simulink model "escestimatorfinal"  (R2021a)
settings: Solver=VariableStepAuto  StartTime=0.0  StopTime=10.0  RelTol=1e-3
values from neighbouring files (symbols this model uses):
  B = 18    [fourwheelvdmodelparam.m]
  C = 1.5    [fourwheelvdmodelparam.m]
  C_A = 0.5    [fourwheelvdmodelparam.m]
  Cr = 5800    [fourwheelvdmodelparam.m]
  Cy = 95000    [fourwheelvdmodelparam.m]
  D = 2000    [fourwheelvdmodelparam.m]
  g = 9.81    [fourwheelvdmodelparam.m]
  hs = 0.5    [fourwheelvdmodelparam.m]
  J = (0.5*(lf+lr))^2*m    (= 3825)    [fourwheelvdmodelparam.m]
  Jx = 800    [fourwheelvdmodelparam.m]
  K = 42000    [fourwheelvdmodelparam.m]
  lf = 1.5    [fourwheelvdmodelparam.m]
  lr = 1.5    [fourwheelvdmodelparam.m]
  m = 1700    [fourwheelvdmodelparam.m]
undefined symbols (not defined in the file or in its folder): Cx, Sfl, Sfr, Srl, Srr
libraries: simulink x2
settings Model: Creator=s361515  LastModifiedBy=s361515

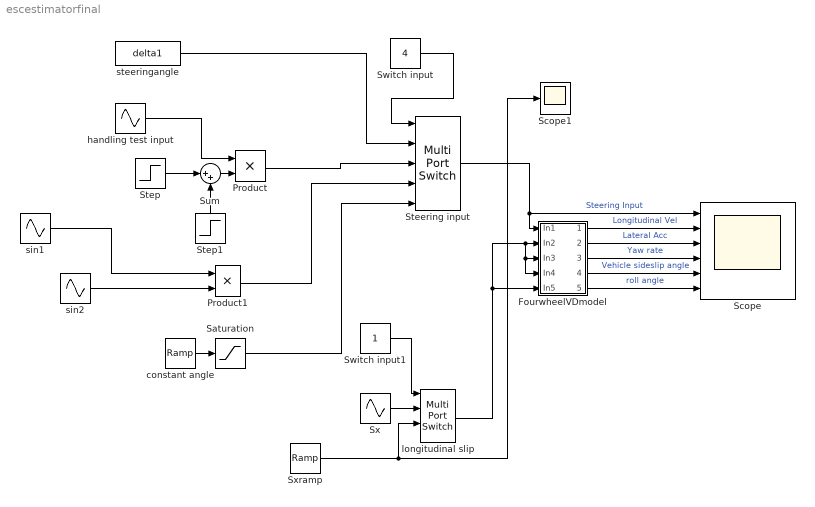
== system escestimatorfinal ==
  FourwheelVDmodel : Subsystem
  Product : Product
  Product1 : Product
  Saturation : Saturate  UpperLimit=5  LowerLimit=0
  Scope : Scope  NumInputPorts=6
  Scope1 : Scope
  Steering input : MultiPortSwitch  Inputs=4
  Step : Step  Time=1.5  SampleTime=0
  Step1 : Step  Time=8.5  After=-1  SampleTime=0
  Sum : Sum  Inputs=|++
  Switch input : Constant  Value=4
  Switch input1 : Constant
  Sx : Sin  Amplitude=0.5e-1  Bias=1.5e-1  Frequency=5*pi  SampleTime=0
  Sxramp : simulink/Sources/Ramp  slope=0.1  start=0  InitialOutput=0
  constant angle : simulink/Sources/Ramp  slope=1.5  start=0  InitialOutput=0
  handling test input : Sin  Amplitude=6  Frequency=pi  Phase=pi/2  SampleTime=0
  longitudinal slip : MultiPortSwitch
  sin1 : Sin  Amplitude=6  Frequency=pi/8  SampleTime=0
  sin2 : Sin  Frequency=pi  Phase=pi/2  SampleTime=0
  steeringangle : FromWorkspace  VariableName=delta1
  wires:
  sin1/1 -> Product1/1
  Product1/1 -> Steering input/4
  longitudinal slip/1 -> FourwheelVDmodel/5(In5), FourwheelVDmodel/4(In4), FourwheelVDmodel/3(In3), FourwheelVDmodel/2(In2)
  Switch input1/1 -> longitudinal slip/1
  Sxramp/1 -> Scope1/1, longitudinal slip/3
  sin2/1 -> Product1/2
  Step/1 -> Sum/1
  Step1/1 -> Sum/2
  handling test input/1 -> Product/1
  FourwheelVDmodel/1(Out1) -> Scope/2  "Longitudinal Vel"
  Product/1 -> Steering input/3
  FourwheelVDmodel/2(Out2) -> Scope/3  "Lateral Acc"
  Steering input/1 -> FourwheelVDmodel/1(In1), Scope/1  "Steering Input"
  Sum/1 -> Product/2
  constant angle/1 -> Saturation/1
  Sx/1 -> longitudinal slip/2
  FourwheelVDmodel/3(Out3) -> Scope/4  "Yaw rate"
  Switch input/1 -> Steering input/1
  FourwheelVDmodel/5(Out5) -> Scope/6  "roll angle"
  FourwheelVDmodel/4(Out4) -> Scope/5  "Vehicle sideslip angle"
  Saturation/1 -> Steering input/5
  steeringangle/1 -> Steering input/2

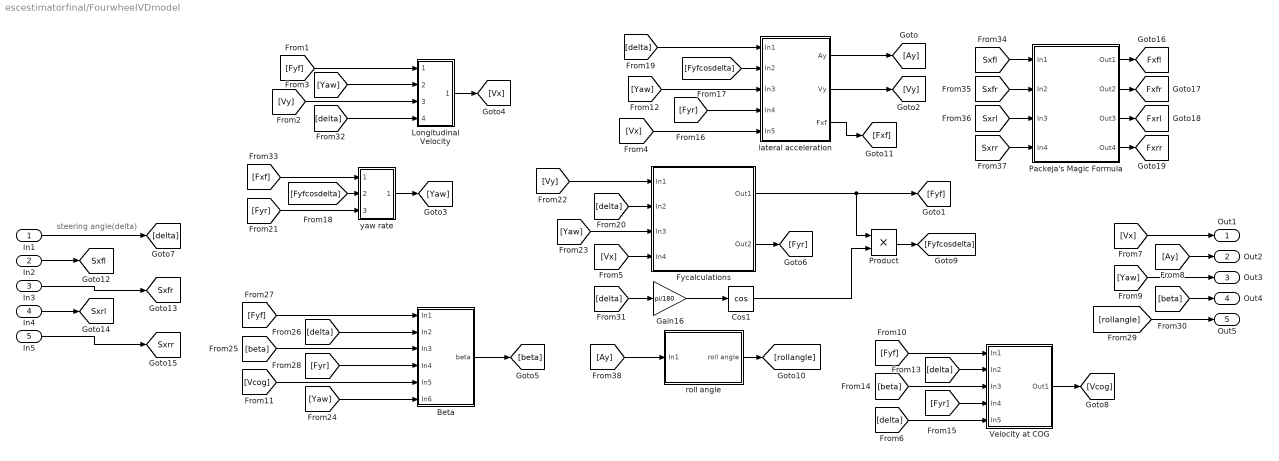
== system escestimatorfinal/FourwheelVDmodel ==
  note: steering angle(delta)
  In1 : Inport
  In2 : Inport  Port=2
  In3 : Inport  Port=3
  In4 : Inport  Port=4
  In5 : Inport  Port=5
  Beta : Subsystem
  Cos1 : Trigonometry  Operator=cos
  Fycalculations : Subsystem
  Gain16 : Gain  Gain=pi/180
  Longitudinal Velocity : Subsystem
  Packeja's Magic Formula : Subsystem
  Product : Product
  Velocity at COG : Subsystem
  lateral acceleration : Subsystem
  roll angle : Subsystem
  yaw rate : Subsystem
  Out1 : Outport
  Out2 : Outport  Port=2
  Out3 : Outport  Port=3
  Out4 : Outport  Port=4
  Out5 : Outport  Port=5
  tag scope: Fxfl=global, Fxfr=global, Fxrl=global, Fxrr=global, Sxfl=global, Sxfr=global, Sxrl=global, Sxrr=global
  wires:
  Gain16/1 -> Cos1/1
  Product/1 -> [Fyfcosdelta]
  In1/1 -> [delta]
  Cos1/1 -> Product/2
  [Vx] -> Out1/1
  [Ay] -> Out2/1
  [Yaw] -> Out3/1
  Longitudinal Velocity/1(Out1) -> [Vx]
  [Fyf] -> Longitudinal Velocity/1(In1)
  [Yaw] -> Longitudinal Velocity/2(In2)
  [Vy] -> Longitudinal Velocity/3(In3)
  lateral acceleration/2(Vy) -> [Vy]
  [Vx] -> lateral acceleration/5(In5)
  lateral acceleration/1(Ay) -> [Ay]
  [Yaw] -> lateral acceleration/3(In3)
  [Fyr] -> lateral acceleration/4(In4)
  [Fyfcosdelta] -> lateral acceleration/2(In2)
  [delta] -> lateral acceleration/1(In1)
  yaw rate/1(Out1) -> [Yaw]
  [Fyfcosdelta] -> yaw rate/2(In2)
  [Fyr] -> yaw rate/3(In3)
  Fycalculations/1(Out1) -> [Fyf], Product/1
  Fycalculations/2(Out2) -> [Fyr]
  [Vy] -> Fycalculations/1(In1)
  [delta] -> Fycalculations/2(In2)
  [Yaw] -> Fycalculations/3(In3)
  [Vx] -> Fycalculations/4(In4)
  Beta/1(beta) -> [beta]
  [Fyf] -> Beta/1(In1)
  [delta] -> Beta/2(In2)
  [beta] -> Beta/3(In3)
  [Fyr] -> Beta/4(In4)
  [Vcog] -> Beta/5(In5)
  [Yaw] -> Beta/6(In6)
  [Ay] -> roll angle/1(In1)
  roll angle/1(roll angle) -> [rollangle]
  [rollangle] -> Out5/1
  [beta] -> Out4/1
  [Fyf] -> Velocity at COG/1(In1)
  [delta] -> Velocity at COG/2(In2)
  [beta] -> Velocity at COG/3(In3)
  [Fyr] -> Velocity at COG/4(In4)
  [delta] -> Velocity at COG/5(In5)
  Velocity at COG/1(Out1) -> [Vcog]
  [delta] -> Gain16/1
  [delta] -> Longitudinal Velocity/4(In4)
  lateral acceleration/3(Fxf) -> [Fxf]
  [Fxf] -> yaw rate/1(In1)
  In5/1 -> [Sxrr]
  In4/1 -> [Sxrl]
  In3/1 -> [Sxfr]
  In2/1 -> [Sxfl]
  [Sxfl] -> Packeja's Magic Formula/1(In1)
  [Sxfr] -> Packeja's Magic Formula/2(In2)
  [Sxrl] -> Packeja's Magic Formula/3(In3)
  [Sxrr] -> Packeja's Magic Formula/4(In4)
  Packeja's Magic Formula/1(Out1) -> [Fxfl]
  Packeja's Magic Formula/4(Out4) -> [Fxrr]
  Packeja's Magic Formula/3(Out3) -> [Fxrl]
  Packeja's Magic Formula/2(Out2) -> [Fxfr]

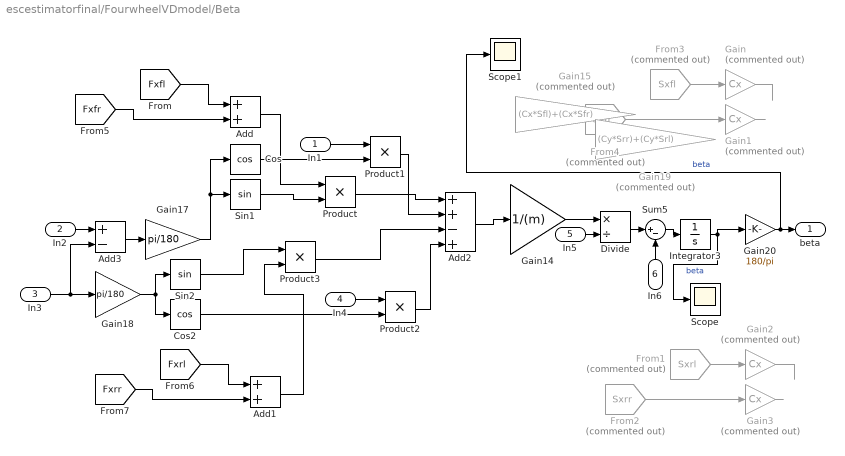
== system escestimatorfinal/FourwheelVDmodel/Beta ==
  In1 : Inport
  In2 : Inport  Port=2
  In3 : Inport  Port=3
  In4 : Inport  Port=4
  In5 : Inport  Port=5
  In6 : Inport  Port=6
  Add : Sum
  Add1 : Sum
  Add2 : Sum  Inputs=++-+
  Add3 : Sum  Inputs=+-
  Cos : Trigonometry  Operator=cos
  Cos2 : Trigonometry  Operator=cos
  Divide : Product  Inputs=*/
  From1 : From  Commented=on  GotoTag=Sxrl  TagVisibility=global
  From2 : From  Commented=on  GotoTag=Sxrr  TagVisibility=global
  From3 : From  Commented=on  GotoTag=Sxfl  TagVisibility=global
  From4 : From  Commented=on  GotoTag=Sxfr  TagVisibility=global
  Gain{,1..3} (4 alike) : Gain  Commented=on  Gain=Cx
  Gain14 : Gain  Gain=1/(m)
  Gain15 : Gain  Commented=on  Gain=(Cx*Sfl)+(Cx*Sfr)
  Gain17 : Gain  Gain=pi/180
  Gain18 : Gain  Gain=pi/180
  Gain19 : Gain  Commented=on  Gain=(Cy*Srr)+(Cy*Srl)
  Gain20 : Gain  Gain=180/pi
  Integrator3 : Integrator
  Product{,1..3} (4 alike) : Product
  Scope : Scope
  Scope1 : Scope
  Sin1 : Trigonometry
  Sin2 : Trigonometry
  Sum5 : Sum  Inputs=|+-
  beta : Outport
  wires:
  Product1/1 -> Add2/2
  Product/1 -> Add2/1
  Sin1/1 -> Product/2
  In3/1 -> Gain18/1, Add3/2
  In1/1 -> Product1/1
  Gain18/1 -> Sin2/1, Cos2/1
  Cos2/1 -> Product2/2
  Gain17/1 -> Cos/1, Sin1/1
  Integrator3/1 -> Gain20/1, Scope/1  "beta"
  In6/1 -> Sum5/2
  Sum5/1 -> Integrator3/1
  Cos/1 -> Product1/2
  Add2/1 -> Gain14/1
  Sin2/1 -> Product3/1
  Gain14/1 -> Divide/1
  In5/1 -> Divide/2
  Add3/1 -> Gain17/1
  Gain20/1 -> Scope1/1, beta/1  "beta"
  In2/1 -> Add3/1
  Divide/1 -> Sum5/1
  Product3/1 -> Add2/3
  In4/1 -> Product2/1
  From3/1 -> Gain/1
  From4/1 -> Gain1/1
  Add/1 -> Product/1
  Gain1/1 -> ?
  Gain/1 -> ?
  From1/1 -> Gain2/1
  From2/1 -> Gain3/1
  Add1/1 -> Product3/2
  Gain3/1 -> ?
  Gain2/1 -> ?
  [Fxfl] -> Add/1
  [Fxfr] -> Add/2
  [Fxrl] -> Add1/1
  [Fxrr] -> Add1/2
  Product2/1 -> Add2/4

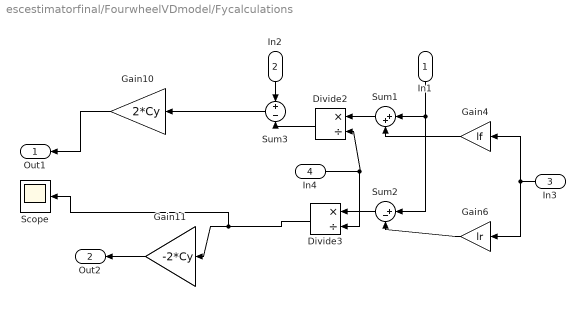
== system escestimatorfinal/FourwheelVDmodel/Fycalculations ==
  In1 : Inport
  In2 : Inport  Port=2
  In3 : Inport  Port=3
  In4 : Inport  Port=4
  Divide2 : Product  Inputs=*/
  Divide3 : Product  Inputs=*/
  Gain10 : Gain  Gain=2*Cy
  Gain11 : Gain  Gain=-2*Cy
  Gain4 : Gain  Gain=lf
  Gain6 : Gain  Gain=lr
  Scope : Scope
  Sum1 : Sum  Inputs=|++
  Sum2 : Sum  Inputs=|+-
  Sum3 : Sum  Inputs=+-
  Out1 : Outport
  Out2 : Outport  Port=2
  wires:
  Gain4/1 -> Sum1/2
  Sum3/1 -> Gain10/1
  Gain6/1 -> Sum2/2
  In4/1 -> Divide3/2, Divide2/2
  Divide2/1 -> Sum3/2
  Sum1/1 -> Divide2/1
  Sum2/1 -> Divide3/1
  In3/1 -> Gain4/1, Gain6/1
  In1/1 -> Sum1/1, Sum2/1
  In2/1 -> Sum3/1
  Gain11/1 -> Out2/1
  Gain10/1 -> Out1/1
  Divide3/1 -> Scope/1, Gain11/1

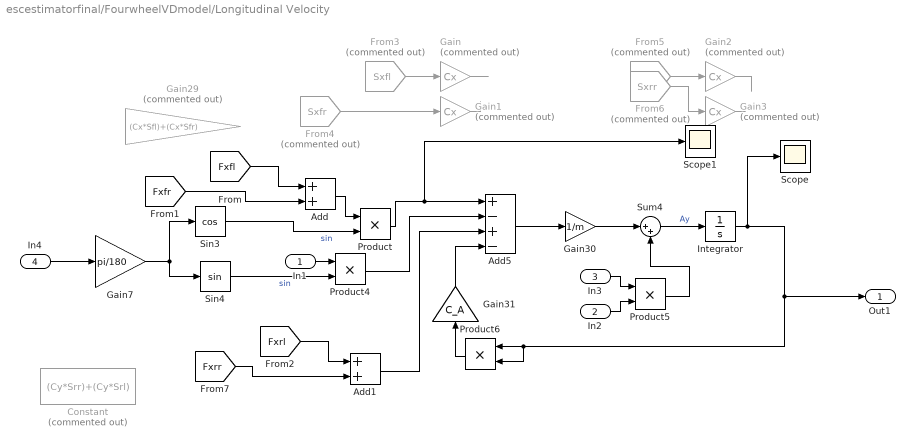
== system escestimatorfinal/FourwheelVDmodel/Longitudinal Velocity ==
  In1 : Inport
  In2 : Inport  Port=2
  In3 : Inport  Port=3
  In4 : Inport  Port=4
  Add : Sum
  Add1 : Sum
  Add5 : Sum  Inputs=+-+-
  Constant : Constant  Commented=on  Value=(Cy*Srr)+(Cy*Srl)
  From3 : From  Commented=on  GotoTag=Sxfl  TagVisibility=global
  From4 : From  Commented=on  GotoTag=Sxfr  TagVisibility=global
  From5 : From  Commented=on  GotoTag=Sxrl  TagVisibility=global
  From6 : From  Commented=on  GotoTag=Sxrr  TagVisibility=global
  Gain{,1..3} (4 alike) : Gain  Commented=on  Gain=Cx
  Gain29 : Gain  Commented=on  Gain=(Cx*Sfl)+(Cx*Sfr)
  Gain30 : Gain  Gain=1/m
  Gain31 : Gain  Gain=C_A
  Gain7 : Gain  Gain=pi/180
  Integrator : Integrator  InitialCondition=20
  Product{,4..6} (4 alike) : Product
  Scope : Scope
  Scope1 : Scope
  Sin3 : Trigonometry  Operator=cos
  Sin4 : Trigonometry
  Sum4 : Sum  Inputs=|++
  Out1 : Outport
  wires:
  Gain30/1 -> Sum4/1
  Sin4/1 -> Product4/2  "sin"
  Product/1 -> Scope1/1, Add5/1
  Add5/1 -> Gain30/1
  In1/1 -> Product4/1
  Sum4/1 -> Integrator/1  "Ay"
  Sin3/1 -> Product/2  "sin"
  Gain7/1 -> Sin4/1, Sin3/1
  Product6/1 -> Gain31/1
  Gain31/1 -> Add5/4
  In4/1 -> Gain7/1
  Add1/1 -> Add5/3
  In3/1 -> Product5/1
  Product5/1 -> Sum4/2
  Product4/1 -> Add5/2
  Integrator/1 -> Scope/1, Out1/1, Product6/2, Product6/1
  In2/1 -> Product5/2
  From3/1 -> Gain/1
  From4/1 -> Gain1/1
  Gain/1 -> ?
  Gain1/1 -> ?
  Add/1 -> Product/1
  From5/1 -> Gain2/1
  From6/1 -> Gain3/1
  Gain3/1 -> ?
  Gain2/1 -> ?
  [Fxfl] -> Add/1
  [Fxfr] -> Add/2
  [Fxrl] -> Add1/1
  [Fxrr] -> Add1/2

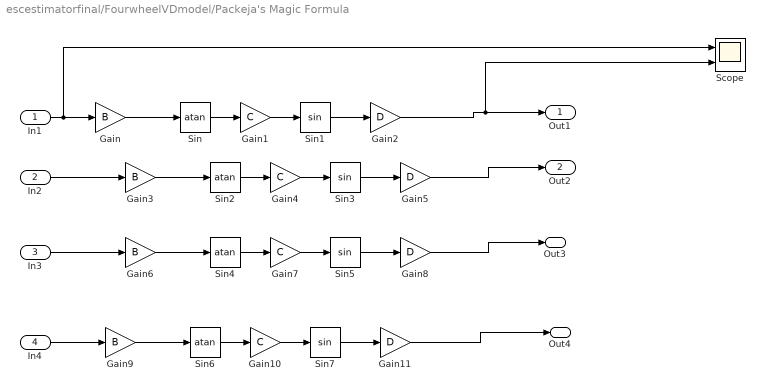
== system escestimatorfinal/FourwheelVDmodel/Packeja's Magic Formula ==
  In1 : Inport
  In2 : Inport  Port=2
  In3 : Inport  Port=3
  In4 : Inport  Port=4
  Gain{,3,6,9} (4 alike) : Gain  Gain=B
  Gain{1,4,7,10} (4 alike) : Gain  Gain=C
  Gain{2,5,8,11} (4 alike) : Gain  Gain=D
  Scope : Scope  NumInputPorts=2
  Sin{,2,4,6} (4 alike) : Trigonometry  Operator=atan
  Sin{1,3,5,7} (4 alike) : Trigonometry
  Out1 : Outport
  Out2 : Outport  Port=2
  Out3 : Outport  Port=3
  Out4 : Outport  Port=4
  wires:
  In1/1 -> Scope/1, Gain/1
  Sin/1 -> Gain1/1
  Gain/1 -> Sin/1
  Gain1/1 -> Sin1/1
  Sin1/1 -> Gain2/1
  Gain2/1 -> Scope/2, Out1/1
  Gain5/1 -> Out2/1
  Sin3/1 -> Gain5/1
  Gain4/1 -> Sin3/1
  Gain3/1 -> Sin2/1
  Sin2/1 -> Gain4/1
  In2/1 -> Gain3/1
  In3/1 -> Gain6/1
  Sin4/1 -> Gain7/1
  Gain6/1 -> Sin4/1
  Gain7/1 -> Sin5/1
  Sin5/1 -> Gain8/1
  Gain8/1 -> Out3/1
  Gain11/1 -> Out4/1
  Sin7/1 -> Gain11/1
  Gain10/1 -> Sin7/1
  Gain9/1 -> Sin6/1
  Sin6/1 -> Gain10/1
  In4/1 -> Gain9/1

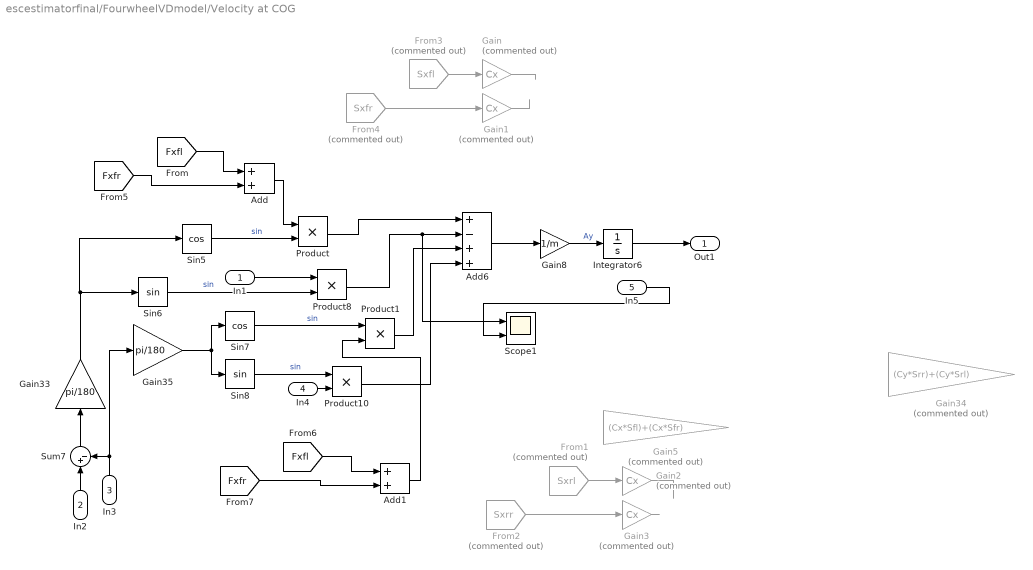
== system escestimatorfinal/FourwheelVDmodel/Velocity at COG ==
  In1 : Inport
  In2 : Inport  Port=2
  In3 : Inport  Port=3
  In4 : Inport  Port=4
  In5 : Inport  Port=5
  Add : Sum
  Add1 : Sum
  Add6 : Sum  Inputs=+-++
  From1 : From  Commented=on  GotoTag=Sxrl  TagVisibility=global
  From2 : From  Commented=on  GotoTag=Sxrr  TagVisibility=global
  From3 : From  Commented=on  GotoTag=Sxfl  TagVisibility=global
  From4 : From  Commented=on  GotoTag=Sxfr  TagVisibility=global
  Gain{,1..3} (4 alike) : Gain  Commented=on  Gain=Cx
  Gain33 : Gain  Gain=pi/180
  Gain34 : Gain  Commented=on  Gain=(Cy*Srr)+(Cy*Srl)
  Gain35 : Gain  Gain=pi/180
  Gain5 : Gain  Commented=on  Gain=(Cx*Sfl)+(Cx*Sfr)
  Gain8 : Gain  Gain=1/m
  Integrator6 : Integrator  InitialCondition=20
  Product{,1,8,10} (4 alike) : Product
  Scope1 : Scope  NumInputPorts=2
  Sin5 : Trigonometry  Operator=cos
  Sin6 : Trigonometry
  Sin7 : Trigonometry  Operator=cos
  Sin8 : Trigonometry
  Sum7 : Sum  Inputs=|+-
  Out1 : Outport
  wires:
  Integrator6/1 -> Out1/1
  Product1/1 -> Add6/3
  Gain35/1 -> Sin8/1, Sin7/1
  Sin5/1 -> Product/2  "sin"
  Product8/1 -> Scope1/1, Add6/2
  Sin7/1 -> Product1/1  "sin"
  Gain8/1 -> Integrator6/1  "Ay"
  Gain33/1 -> Sin5/1, Sin6/1
  Product/1 -> Add6/1
  In5/1 -> Scope1/2
  Add6/1 -> Gain8/1
  Sin8/1 -> Product10/1  "sin"
  In3/1 -> Sum7/2, Gain35/1
  Sin6/1 -> Product8/2  "sin"
  Sum7/1 -> Gain33/1
  Product10/1 -> Add6/4
  In1/1 -> Product8/1
  In2/1 -> Sum7/1
  In4/1 -> Product10/2
  From3/1 -> Gain/1
  From4/1 -> Gain1/1
  Add/1 -> Product/1
  Gain1/1 -> ?
  Gain/1 -> ?
  From1/1 -> Gain2/1
  From2/1 -> Gain3/1
  Add1/1 -> Product1/2
  Gain3/1 -> ?
  Gain2/1 -> ?
  [Fxfl] -> Add/1
  [Fxfr] -> Add/2
  [Fxfl] -> Add1/1
  [Fxfr] -> Add1/2

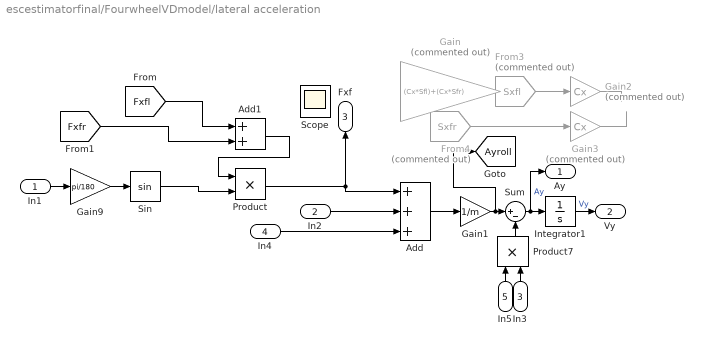
== system escestimatorfinal/FourwheelVDmodel/lateral acceleration ==
  In1 : Inport
  In2 : Inport  Port=2
  In3 : Inport  Port=3
  In4 : Inport  Port=4
  In5 : Inport  Port=5
  Add : Sum  Inputs=+++
  Add1 : Sum
  From3 : From  Commented=on  GotoTag=Sxfl  TagVisibility=global
  From4 : From  Commented=on  GotoTag=Sxfr  TagVisibility=global
  Gain : Gain  Commented=on  Gain=(Cx*Sfl)+(Cx*Sfr)
  Gain1 : Gain  Gain=1/m
  Gain2 : Gain  Commented=on  Gain=Cx
  Gain3 : Gain  Commented=on  Gain=Cx
  Gain9 : Gain  Gain=pi/180
  Integrator1 : Integrator
  Product : Product
  Product7 : Product
  Scope : Scope
  Sin : Trigonometry
  Sum : Sum  Inputs=|+-
  Ay : Outport
  Vy : Outport  Port=2
  Fxf : Outport  Port=3
  tag scope: Ayroll=global
  wires:
  Gain9/1 -> Sin/1
  Gain1/1 -> [Ayroll], Sum/1
  Integrator1/1 -> Vy/1  "Vy"
  Product/1 -> Add/1, Fxf/1
  Product7/1 -> Sum/2
  Add/1 -> Gain1/1
  Sum/1 -> Ay/1, Integrator1/1  "Ay"
  Sin/1 -> Product/2
  In3/1 -> Product7/2
  In2/1 -> Add/2
  In1/1 -> Gain9/1
  In5/1 -> Product7/1
  In4/1 -> Add/3
  From3/1 -> Gain2/1
  From4/1 -> Gain3/1
  Add1/1 -> Product/1
  Gain3/1 -> ?
  Gain2/1 -> ?
  [Fxfl] -> Add1/1
  [Fxfr] -> Add1/2

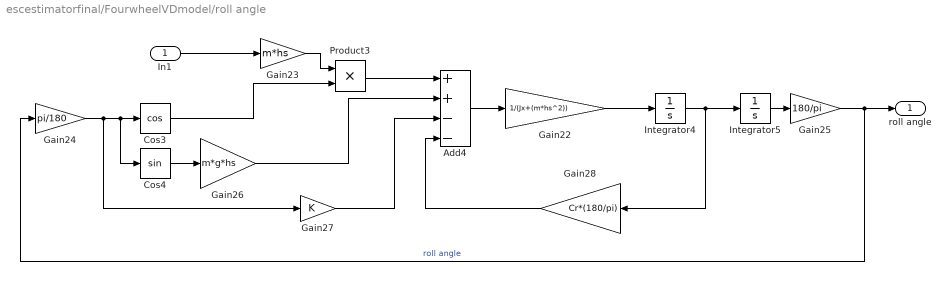
== system escestimatorfinal/FourwheelVDmodel/roll angle ==
  In1 : Inport
  Add4 : Sum  Inputs=++--
  Cos3 : Trigonometry  Operator=cos
  Cos4 : Trigonometry
  Gain22 : Gain  Gain=1/(Jx+(m*hs^2))
  Gain23 : Gain  Gain=m*hs
  Gain24 : Gain  Gain=pi/180
  Gain25 : Gain  Gain=180/pi
  Gain26 : Gain  Gain=m*g*hs
  Gain27 : Gain  Gain=K
  Gain28 : Gain  Gain=Cr*(180/pi)
  Integrator4 : Integrator
  Integrator5 : Integrator
  Product3 : Product
  roll angle : Outport
  wires:
  Cos4/1 -> Gain26/1
  Gain26/1 -> Add4/2
  Integrator4/1 -> Gain28/1, Integrator5/1
  Gain28/1 -> Add4/4
  Product3/1 -> Add4/1
  Cos3/1 -> Product3/2
  Gain22/1 -> Integrator4/1
  Gain24/1 -> Gain27/1, Cos4/1, Cos3/1
  Gain25/1 -> Gain24/1, roll angle/1  "roll angle"
  Add4/1 -> Gain22/1
  Gain27/1 -> Add4/3
  Gain23/1 -> Product3/1
  Integrator5/1 -> Gain25/1
  In1/1 -> Gain23/1

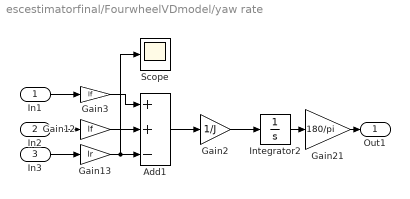
== system escestimatorfinal/FourwheelVDmodel/yaw rate ==
  In1 : Inport
  In2 : Inport  Port=2
  In3 : Inport  Port=3
  Add1 : Sum  Inputs=++-
  Gain12 : Gain  Gain=lf
  Gain13 : Gain  Gain=lr
  Gain2 : Gain  Gain=1/J
  Gain21 : Gain  Gain=180/pi
  Gain3 : Gain  Gain=lf
  Integrator2 : Integrator
  Scope : Scope
  Out1 : Outport
  wires:
  Integrator2/1 -> Gain21/1
  Gain21/1 -> Out1/1
  In3/1 -> Gain13/1
  Gain13/1 -> Scope/1, Add1/3
  Gain12/1 -> Add1/2
  Add1/1 -> Gain2/1
  Gain2/1 -> Integrator2/1
  Gain3/1 -> Add1/1
  In1/1 -> Gain3/1
  In2/1 -> Gain12/1
